simulink model "ConsolidatedModelV9"  (R2022a)
settings: Solver=VariableStepAuto  StartTime=0.0  StopTime=10.0  RelTol=1e-3
undefined symbols (not defined in the file or in its folder): s0
libraries: commblkcod2 x15, commchan3 x12, commdigbbndpm3 x12, simulink x9, commsink2 x6, commdigbbndam3 x6, rllib x3
settings Model: Creator=yangz  LastModifiedBy=yangz

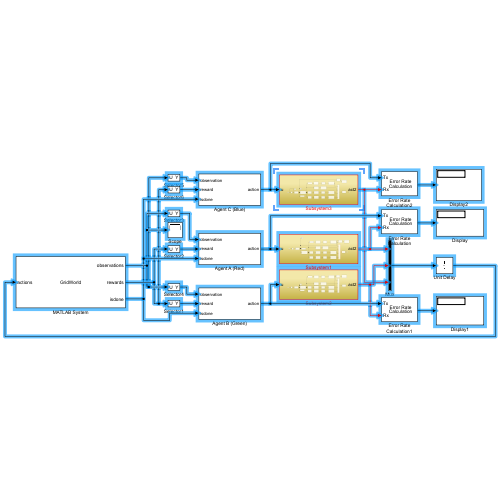
[thumbnail: Simulink's stored preview of the top-level diagram]
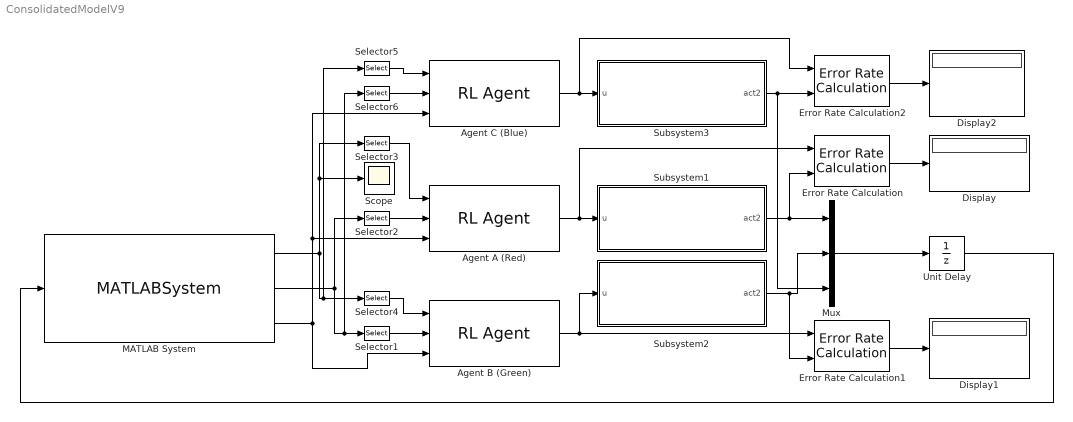
== system ConsolidatedModelV9 ==
  Agent A (Red) : rllib/RL Agent  Agent=agentA  ExternalActionAsInput=off  ProvideLastAction=off  ProvideCumRwd=off  TreatAsDirectFeedthrough=on  UseStrictObservationDataTypes=off
  Agent B (Green) : rllib/RL Agent  Agent=agentB  ExternalActionAsInput=off  ProvideLastAction=off  ProvideCumRwd=off  TreatAsDirectFeedthrough=on  UseStrictObservationDataTypes=off
  Agent C (Blue) : rllib/RL Agent  Agent=agentC  ExternalActionAsInput=off  ProvideLastAction=off  ProvideCumRwd=off  TreatAsDirectFeedthrough=on  UseStrictObservationDataTypes=off
  Display : Display
  Display1 : Display
  Display2 : Display
  Error Rate Calculation : commsink2/Error Rate Calculation  N=0  st_delay=0  cp_mode=Entire frame  subframe=[]  PMode=Port  WsName=ErrorVec  RsMode2=off  stop=off  numErr=100  maxBits=1e6
  Error Rate Calculation1 : commsink2/Error Rate Calculation  N=0  st_delay=0  cp_mode=Entire frame  subframe=[]  PMode=Port  WsName=ErrorVec  RsMode2=off  stop=off  numErr=100  maxBits=1e6
  Error Rate Calculation2 : commsink2/Error Rate Calculation  N=0  st_delay=0  cp_mode=Entire frame  subframe=[]  PMode=Port  WsName=ErrorVec  RsMode2=off  stop=off  numErr=100  maxBits=1e6
  MATLAB System : MATLABSystem  System=GridWorld  InitialStates=s0  Obstacles=obsMat  MaxStepCount=maxsteps  SimulateUsing=Interpreted execution
      mask Type: GridWorld
      mask Display:
      | disp('GridWorld');
      | port_label('input',1,'actions');
      | port_label('output',1,'observations');
      | port_label('output',2,'rewards');
      | port_label('output',3,'isdone');
  Mux : Mux  Inputs=3
  Scope : Scope
  Selector1 : Selector  InputPortWidth=3  IndexOptions=Index vector (dialog)  Indices=2  OutputSizes=1
  Selector2 : Selector  InputPortWidth=3  IndexOptions=Index vector (dialog)  Indices=1  OutputSizes=1
  Selector3 : Selector  NumberOfDimensions=4  InputPortWidth=3  IndexOptions=Select all,Select all,Select all,Index vector (dialog)  Indices=1,1,1,1  OutputSizes=1,1,1,1
  Selector4 : Selector  NumberOfDimensions=4  InputPortWidth=3  IndexOptions=Select all,Select all,Select all,Index vector (dialog)  Indices=1,1,1,2  OutputSizes=1,1,1,1
  Selector5 : Selector  NumberOfDimensions=4  InputPortWidth=3  IndexOptions=Select all,Select all,Select all,Index vector (dialog)  Indices=1,1,1,3  OutputSizes=1,1,1,1
  Selector6 : Selector  InputPortWidth=3  IndexOptions=Index vector (dialog)  Indices=3  OutputSizes=1
  Subsystem1 : Subsystem
  Subsystem2 : Subsystem
  Subsystem3 : Subsystem
  Unit Delay : UnitDelay  SampleTime=-1  HasFrameUpgradeWarning=on
  wires:
  Agent C (Blue)/1 -> Error Rate Calculation2/1, Subsystem3/1(u)
  Mux/1 -> Unit Delay/1
  MATLAB System/1 -> Selector4/1, Selector5/1, Scope/1, Selector3/1
  MATLAB System/3 -> Agent B (Green)/3, Agent A (Red)/3, Agent C (Blue)/3
  MATLAB System/2 -> Selector1/1, Selector6/1, Selector2/1
  Subsystem3/1(act2) -> Mux/3, Error Rate Calculation2/2
  Selector5/1 -> Agent C (Blue)/1
  Error Rate Calculation/1 -> Display/1
  Agent B (Green)/1 -> Subsystem2/1(u), Error Rate Calculation1/1
  Agent A (Red)/1 -> Subsystem1/1(u), Error Rate Calculation/1
  Subsystem2/1(act2) -> Mux/2, Error Rate Calculation1/2
  Subsystem1/1(act2) -> Mux/1, Error Rate Calculation/2
  Selector1/1 -> Agent B (Green)/2
  Selector6/1 -> Agent C (Blue)/2
  Selector4/1 -> Agent B (Green)/1
  Error Rate Calculation2/1 -> Display2/1
  Unit Delay/1 -> MATLAB System/1
  Selector3/1 -> Agent A (Red)/1
  Selector2/1 -> Agent A (Red)/2
  Error Rate Calculation1/1 -> Display1/1

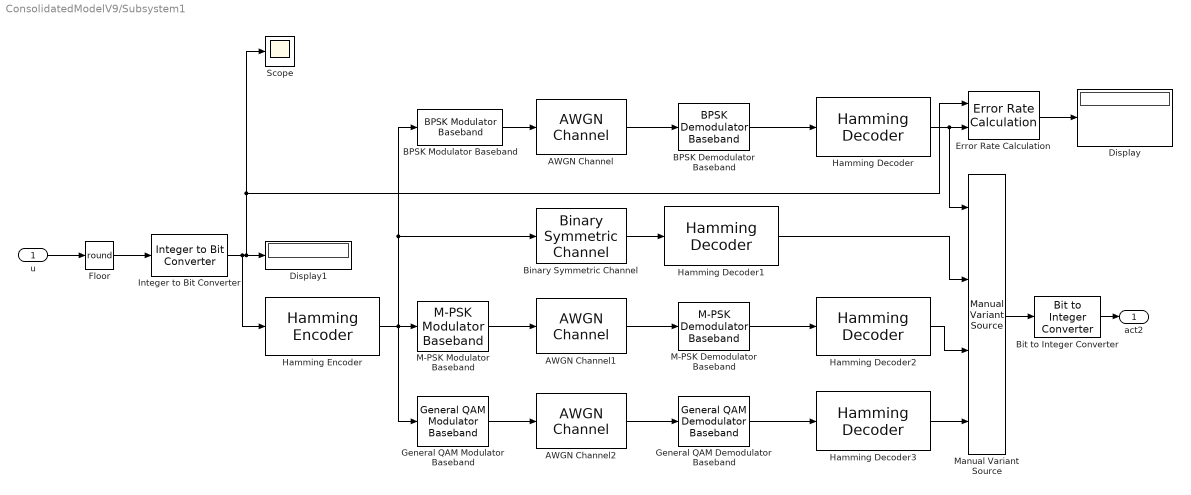
== system ConsolidatedModelV9/Subsystem1 ==
  u : Inport
  AWGN Channel : commchan3/AWGN Channel  InputProcessing=Columns as channels (frame based)  seed=67  noiseMode="Signal to noise ratio  (SNR)"  EbNodB=10  EsNodB=10  SNRdB=10  bitsPerSym=1  Ps=1  Tsym=1  variance=1
  AWGN Channel1 : commchan3/AWGN Channel  InputProcessing=Columns as channels (frame based)  seed=67  noiseMode="Signal to noise ratio  (SNR)"  EbNodB=10  EsNodB=10  SNRdB=10  bitsPerSym=1  Ps=1  Tsym=1  variance=1
  AWGN Channel2 : commchan3/AWGN Channel  InputProcessing=Columns as channels (frame based)  seed=67  noiseMode="Signal to noise ratio  (SNR)"  EbNodB=10  EsNodB=10  SNRdB=10  bitsPerSym=1  Ps=1  Tsym=1  variance=1
  BPSK Demodulator Baseband : commdigbbndpm3/BPSK Demodulator Baseband  DecType=Hard decision  VarSource=Dialog  Variance=1  Ph=0  outDtype=Inherit via internal rule  derotateFactorWordLen=16  derotateFactorDataTypeStr=Inherit: Same word length as input  derotateFactorLastDataTypeStr=Inherit: Same word length as input
  BPSK Modulator Baseband : commdigbbndpm3/BPSK Modulator Baseband  Ph=0  outDtype=double  outWordLen=16  outUDDataType=sfix(16)  outFracLenMode=Best precision  outFracLen=15  outDataTypeStr=double  outLastDataTypeStr=double
  Binary Symmetric Channel : commchan3/Binary Symmetric Channel  ErrorProbability=0.05  ErrorVectorOutputPort=off  OutputDataType=double  OutputDataTypeSL=double  Seed=71  SimulateUsing=Code generation
      settings: SourceProductBaseCode=CM
  Bit to Integer Converter : simulink/Logic and Bit Operations/Bit to Integer Converter  nbits=4  bitOrder=MSB first  signedOutputValues=Unsigned  outDtype=Inherit via internal rule  outDtypeSigned=Inherit via internal rule
      settings: SourceProductBaseCode=SL
  Display : Display
  Display1 : Display
  Error Rate Calculation : commsink2/Error Rate Calculation  N=0  st_delay=0  cp_mode=Entire frame  subframe=[]  PMode=Port  WsName=ErrorVec  RsMode2=off  stop=off  numErr=100  maxBits=1e6
  Floor : Rounding  Operator=round
  General QAM Demodulator Baseband : commdigbbndam3/General QAM Demodulator Baseband  SigCon=[exp(2*pi*1i*[0:7]/8)]  OutType=Integer  DecType=Hard decision  VarSource=Dialog  Variance=1  outDtypeBit=Inherit via internal rule  outDtype=Inherit via internal rule  roundingMode=Floor  overflowMode=Wrap  OvFlMode=off  OvFlModeLastStrValue=off  sigConstWordLen=16  sigConstDataTypeStr=Inherit: Same word length as input  sigConstLastDataTypeStr=Inherit: Same word length as input  accum1WordLen=32  accum1FracLen=30  prodInWordLen=32  prodInFracLen=30  prodInDataTypeStr=Inherit: Same as accumulator 1  prodInLastDataTypeStr=Inherit: Same as accumulator 1  prodOutWordLen=32  prodOutFracLen=30  accum2WordLen=32  accum2FracLen=30  accum3WordLen=32  accum3FracLen=30  nsiWordLen=32  nsiFracLen=30  nsiDataTypeStr=Inherit: Same as accumulator 3  nsiLastDataTypeStr=Inherit: Same as accumulator 3  invn0WordLen=16  invn0FracLen=8  invn0DataTypeStr=Inherit: Same word length as input  invn0LastDataTypeStr=Inherit: Same word length as input  outputWordLen=32  outputFracLen=30
      settings: SourceProductBaseCode=CM
  General QAM Modulator Baseband : commdigbbndam3/General QAM Modulator Baseband  SigCon=[exp(2*pi*1i*[0:7]/8)]  outDtype=double  outWordLen=16  outUDDataType=sfix(16)  outFracLenMode=Best precision  outFracLen=15  outDataTypeStr=double  outLastDataTypeStr=double
      settings: SourceProductBaseCode=CM
  Hamming Decoder{,1..3} (4 alike) : commblkcod2/Hamming Decoder  n=7  k=4
      settings: SourceProductBaseCode=CM
  Hamming Encoder : commblkcod2/Hamming Encoder  n=7  k=4
      settings: SourceProductBaseCode=CM
  Integer to Bit Converter : simulink/Logic and Bit Operations/Integer to Bit Converter  nbits=4  signedInputValues=Unsigned  bitOrder=MSB first  outDtype=Inherit via internal rule
      settings: SourceProductBaseCode=SL
  M-PSK Demodulator Baseband : commdigbbndpm3/M-PSK Demodulator Baseband  M=8  OutType=Integer  DecType=Hard decision  VarSource=Dialog  Variance=1  Dec=Gray  Mapping=[0:7]  Ph=pi/8  outDtype1=Inherit via internal rule  outDtype2=Inherit via internal rule  derotateFactorWordLen=16  derotateFactorDataTypeStr=Inherit: Same word length as input  derotateFactorLastDataTypeStr=Inherit: Same word length as input
  M-PSK Modulator Baseband : commdigbbndpm3/M-PSK Modulator Baseband  M=8  InType=Integer  Enc=Gray  Mapping=[0:7]  Ph=pi/8  outDtype=double  outWordLen=16  outUDDataType=sfix(16)  outFracLenMode=Best precision  outFracLen=15  outDataTypeStr=double  outLastDataTypeStr=double
  Manual Variant Source : simulink/Signal Routing/Manual Variant Source  NumChoices=4  LabelModeActiveChoice=V_3
  Scope : Scope
  act2 : Outport
  wires:
  Binary Symmetric Channel/1 -> Hamming Decoder1/1
  AWGN Channel1/1 -> M-PSK Demodulator Baseband/1
  BPSK Demodulator Baseband/1 -> Hamming Decoder/1
  M-PSK Demodulator Baseband/1 -> Hamming Decoder2/1
  M-PSK Modulator Baseband/1 -> AWGN Channel1/1
  Error Rate Calculation/1 -> Display/1
  AWGN Channel/1 -> BPSK Demodulator Baseband/1
  BPSK Modulator Baseband/1 -> AWGN Channel/1
  Bit to Integer Converter/1 -> act2/1
  General QAM Modulator Baseband/1 -> AWGN Channel2/1
  Floor/1 -> Integer to Bit Converter/1
  u/1 -> Floor/1
  Hamming Decoder1/1 -> Manual Variant Source/2
  AWGN Channel2/1 -> General QAM Demodulator Baseband/1
  Hamming Decoder2/1 -> Manual Variant Source/3
  Hamming Decoder3/1 -> Manual Variant Source/4
  General QAM Demodulator Baseband/1 -> Hamming Decoder3/1
  Hamming Decoder/1 -> Error Rate Calculation/2, Manual Variant Source/1
  Hamming Encoder/1 -> BPSK Modulator Baseband/1, Binary Symmetric Channel/1, M-PSK Modulator Baseband/1, General QAM Modulator Baseband/1
  Integer to Bit Converter/1 -> Error Rate Calculation/1, Scope/1, Display1/1, Hamming Encoder/1
  Manual Variant Source/1 -> Bit to Integer Converter/1

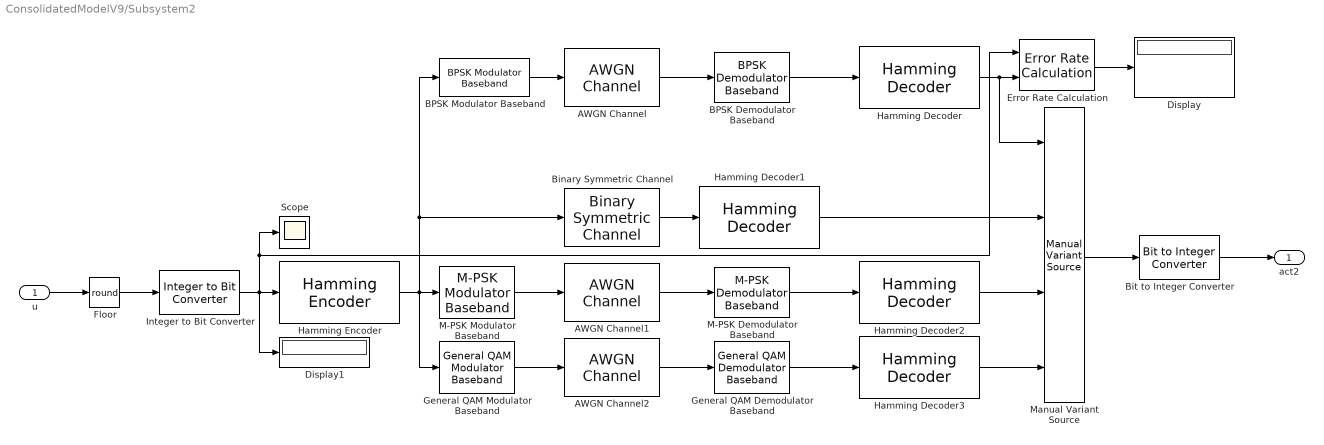
== system ConsolidatedModelV9/Subsystem2 ==
  u : Inport
  AWGN Channel : commchan3/AWGN Channel  InputProcessing=Columns as channels (frame based)  seed=67  noiseMode="Signal to noise ratio  (SNR)"  EbNodB=10  EsNodB=10  SNRdB=10  bitsPerSym=1  Ps=1  Tsym=1  variance=1
  AWGN Channel1 : commchan3/AWGN Channel  InputProcessing=Columns as channels (frame based)  seed=67  noiseMode="Signal to noise ratio  (SNR)"  EbNodB=10  EsNodB=10  SNRdB=10  bitsPerSym=1  Ps=1  Tsym=1  variance=1
  AWGN Channel2 : commchan3/AWGN Channel  InputProcessing=Columns as channels (frame based)  seed=67  noiseMode="Signal to noise ratio  (SNR)"  EbNodB=10  EsNodB=10  SNRdB=10  bitsPerSym=1  Ps=1  Tsym=1  variance=1
  BPSK Demodulator Baseband : commdigbbndpm3/BPSK Demodulator Baseband  DecType=Hard decision  VarSource=Dialog  Variance=1  Ph=0  outDtype=Inherit via internal rule  derotateFactorWordLen=16  derotateFactorDataTypeStr=Inherit: Same word length as input  derotateFactorLastDataTypeStr=Inherit: Same word length as input
  BPSK Modulator Baseband : commdigbbndpm3/BPSK Modulator Baseband  Ph=0  outDtype=double  outWordLen=16  outUDDataType=sfix(16)  outFracLenMode=Best precision  outFracLen=15  outDataTypeStr=double  outLastDataTypeStr=double
  Binary Symmetric Channel : commchan3/Binary Symmetric Channel  ErrorProbability=0.05  ErrorVectorOutputPort=off  OutputDataType=double  OutputDataTypeSL=double  Seed=71  SimulateUsing=Code generation
      settings: SourceProductBaseCode=CM
  Bit to Integer Converter : simulink/Logic and Bit Operations/Bit to Integer Converter  nbits=4  bitOrder=MSB first  signedOutputValues=Unsigned  outDtype=Inherit via internal rule  outDtypeSigned=Inherit via internal rule
      settings: SourceProductBaseCode=SL
  Display : Display
  Display1 : Display
  Error Rate Calculation : commsink2/Error Rate Calculation  N=0  st_delay=0  cp_mode=Entire frame  subframe=[]  PMode=Port  WsName=ErrorVec  RsMode2=off  stop=off  numErr=100  maxBits=1e6
  Floor : Rounding  Operator=round
  General QAM Demodulator Baseband : commdigbbndam3/General QAM Demodulator Baseband  SigCon=[exp(2*pi*1i*[0:7]/8)]  OutType=Integer  DecType=Hard decision  VarSource=Dialog  Variance=1  outDtypeBit=Inherit via internal rule  outDtype=Inherit via internal rule  roundingMode=Floor  overflowMode=Wrap  OvFlMode=off  OvFlModeLastStrValue=off  sigConstWordLen=16  sigConstDataTypeStr=Inherit: Same word length as input  sigConstLastDataTypeStr=Inherit: Same word length as input  accum1WordLen=32  accum1FracLen=30  prodInWordLen=32  prodInFracLen=30  prodInDataTypeStr=Inherit: Same as accumulator 1  prodInLastDataTypeStr=Inherit: Same as accumulator 1  prodOutWordLen=32  prodOutFracLen=30  accum2WordLen=32  accum2FracLen=30  accum3WordLen=32  accum3FracLen=30  nsiWordLen=32  nsiFracLen=30  nsiDataTypeStr=Inherit: Same as accumulator 3  nsiLastDataTypeStr=Inherit: Same as accumulator 3  invn0WordLen=16  invn0FracLen=8  invn0DataTypeStr=Inherit: Same word length as input  invn0LastDataTypeStr=Inherit: Same word length as input  outputWordLen=32  outputFracLen=30
      settings: SourceProductBaseCode=CM
  General QAM Modulator Baseband : commdigbbndam3/General QAM Modulator Baseband  SigCon=[exp(2*pi*1i*[0:7]/8)]  outDtype=double  outWordLen=16  outUDDataType=sfix(16)  outFracLenMode=Best precision  outFracLen=15  outDataTypeStr=double  outLastDataTypeStr=double
      settings: SourceProductBaseCode=CM
  Hamming Decoder{,1..3} (4 alike) : commblkcod2/Hamming Decoder  n=7  k=4
      settings: SourceProductBaseCode=CM
  Hamming Encoder : commblkcod2/Hamming Encoder  n=7  k=4
      settings: SourceProductBaseCode=CM
  Integer to Bit Converter : simulink/Logic and Bit Operations/Integer to Bit Converter  nbits=4  signedInputValues=Unsigned  bitOrder=MSB first  outDtype=Inherit via internal rule
      settings: SourceProductBaseCode=SL
  M-PSK Demodulator Baseband : commdigbbndpm3/M-PSK Demodulator Baseband  M=8  OutType=Integer  DecType=Hard decision  VarSource=Dialog  Variance=1  Dec=Gray  Mapping=[0:7]  Ph=pi/8  outDtype1=Inherit via internal rule  outDtype2=Inherit via internal rule  derotateFactorWordLen=16  derotateFactorDataTypeStr=Inherit: Same word length as input  derotateFactorLastDataTypeStr=Inherit: Same word length as input
  M-PSK Modulator Baseband : commdigbbndpm3/M-PSK Modulator Baseband  M=8  InType=Integer  Enc=Gray  Mapping=[0:7]  Ph=pi/8  outDtype=double  outWordLen=16  outUDDataType=sfix(16)  outFracLenMode=Best precision  outFracLen=15  outDataTypeStr=double  outLastDataTypeStr=double
  Manual Variant Source : simulink/Signal Routing/Manual Variant Source  NumChoices=4  LabelModeActiveChoice=V_3
  Scope : Scope
  act2 : Outport
  wires:
  Manual Variant Source/1 -> Bit to Integer Converter/1
  General QAM Modulator Baseband/1 -> AWGN Channel2/1
  Hamming Decoder1/1 -> Manual Variant Source/2
  Hamming Decoder2/1 -> Manual Variant Source/3
  Hamming Decoder3/1 -> Manual Variant Source/4
  AWGN Channel2/1 -> General QAM Demodulator Baseband/1
  General QAM Demodulator Baseband/1 -> Hamming Decoder3/1
  Floor/1 -> Integer to Bit Converter/1
  M-PSK Demodulator Baseband/1 -> Hamming Decoder2/1
  u/1 -> Floor/1
  Bit to Integer Converter/1 -> act2/1
  M-PSK Modulator Baseband/1 -> AWGN Channel1/1
  Error Rate Calculation/1 -> Display/1
  AWGN Channel/1 -> BPSK Demodulator Baseband/1
  BPSK Demodulator Baseband/1 -> Hamming Decoder/1
  BPSK Modulator Baseband/1 -> AWGN Channel/1
  Binary Symmetric Channel/1 -> Hamming Decoder1/1
  AWGN Channel1/1 -> M-PSK Demodulator Baseband/1
  Hamming Encoder/1 -> Binary Symmetric Channel/1, BPSK Modulator Baseband/1, M-PSK Modulator Baseband/1, General QAM Modulator Baseband/1
  Integer to Bit Converter/1 -> Scope/1, Error Rate Calculation/1, Display1/1, Hamming Encoder/1
  Hamming Decoder/1 -> Manual Variant Source/1, Error Rate Calculation/2

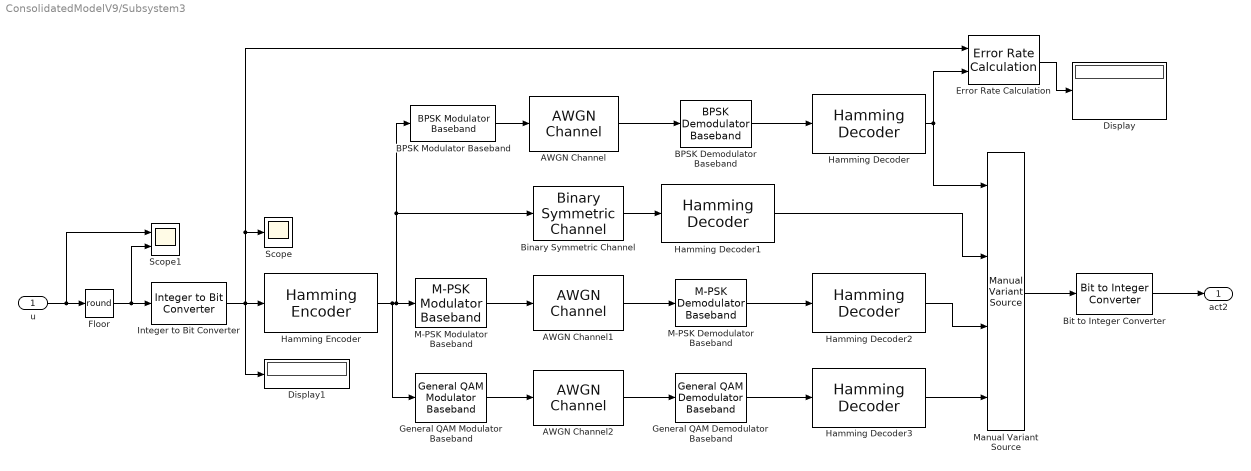
== system ConsolidatedModelV9/Subsystem3 ==
  u : Inport
  AWGN Channel : commchan3/AWGN Channel  InputProcessing=Columns as channels (frame based)  seed=67  noiseMode="Signal to noise ratio  (SNR)"  EbNodB=10  EsNodB=10  SNRdB=10  bitsPerSym=1  Ps=1  Tsym=1  variance=1
  AWGN Channel1 : commchan3/AWGN Channel  InputProcessing=Columns as channels (frame based)  seed=67  noiseMode="Signal to noise ratio  (SNR)"  EbNodB=10  EsNodB=10  SNRdB=10  bitsPerSym=1  Ps=1  Tsym=1  variance=1
  AWGN Channel2 : commchan3/AWGN Channel  InputProcessing=Columns as channels (frame based)  seed=67  noiseMode="Signal to noise ratio  (SNR)"  EbNodB=10  EsNodB=10  SNRdB=10  bitsPerSym=1  Ps=1  Tsym=1  variance=1
  BPSK Demodulator Baseband : commdigbbndpm3/BPSK Demodulator Baseband  DecType=Hard decision  VarSource=Dialog  Variance=1  Ph=0  outDtype=Inherit via internal rule  derotateFactorWordLen=16  derotateFactorDataTypeStr=Inherit: Same word length as input  derotateFactorLastDataTypeStr=Inherit: Same word length as input
  BPSK Modulator Baseband : commdigbbndpm3/BPSK Modulator Baseband  Ph=0  outDtype=double  outWordLen=16  outUDDataType=sfix(16)  outFracLenMode=Best precision  outFracLen=15  outDataTypeStr=double  outLastDataTypeStr=double
  Binary Symmetric Channel : commchan3/Binary Symmetric Channel  ErrorProbability=0.05  ErrorVectorOutputPort=off  OutputDataType=double  OutputDataTypeSL=double  Seed=67  SimulateUsing=Code generation
      settings: SourceProductBaseCode=CM
  Bit to Integer Converter : simulink/Logic and Bit Operations/Bit to Integer Converter  nbits=4  bitOrder=MSB first  signedOutputValues=Unsigned  outDtype=Inherit via internal rule  outDtypeSigned=Inherit via internal rule
      settings: SourceProductBaseCode=SL
  Display : Display
  Display1 : Display
  Error Rate Calculation : commsink2/Error Rate Calculation  N=0  st_delay=0  cp_mode=Entire frame  subframe=[]  PMode=Port  WsName=ErrorVec  RsMode2=off  stop=off  numErr=100  maxBits=1e6
  Floor : Rounding  Operator=round
  General QAM Demodulator Baseband : commdigbbndam3/General QAM Demodulator Baseband  SigCon=[exp(2*pi*1i*[0:7]/8)]  OutType=Integer  DecType=Hard decision  VarSource=Dialog  Variance=1  outDtypeBit=Inherit via internal rule  outDtype=Inherit via internal rule  roundingMode=Floor  overflowMode=Wrap  OvFlMode=off  OvFlModeLastStrValue=off  sigConstWordLen=16  sigConstDataTypeStr=Inherit: Same word length as input  sigConstLastDataTypeStr=Inherit: Same word length as input  accum1WordLen=32  accum1FracLen=30  prodInWordLen=32  prodInFracLen=30  prodInDataTypeStr=Inherit: Same as accumulator 1  prodInLastDataTypeStr=Inherit: Same as accumulator 1  prodOutWordLen=32  prodOutFracLen=30  accum2WordLen=32  accum2FracLen=30  accum3WordLen=32  accum3FracLen=30  nsiWordLen=32  nsiFracLen=30  nsiDataTypeStr=Inherit: Same as accumulator 3  nsiLastDataTypeStr=Inherit: Same as accumulator 3  invn0WordLen=16  invn0FracLen=8  invn0DataTypeStr=Inherit: Same word length as input  invn0LastDataTypeStr=Inherit: Same word length as input  outputWordLen=32  outputFracLen=30
      settings: SourceProductBaseCode=CM
  General QAM Modulator Baseband : commdigbbndam3/General QAM Modulator Baseband  SigCon=[exp(2*pi*1i*[0:7]/8)]  outDtype=double  outWordLen=16  outUDDataType=sfix(16)  outFracLenMode=Best precision  outFracLen=15  outDataTypeStr=double  outLastDataTypeStr=double
      settings: SourceProductBaseCode=CM
  Hamming Decoder{,1..3} (4 alike) : commblkcod2/Hamming Decoder  n=7  k=4
      settings: SourceProductBaseCode=CM
  Hamming Encoder : commblkcod2/Hamming Encoder  n=7  k=4
      settings: SourceProductBaseCode=CM
  Integer to Bit Converter : simulink/Logic and Bit Operations/Integer to Bit Converter  nbits=4  signedInputValues=Unsigned  bitOrder=MSB first  outDtype=Inherit via internal rule
      settings: SourceProductBaseCode=SL
  M-PSK Demodulator Baseband : commdigbbndpm3/M-PSK Demodulator Baseband  M=8  OutType=Integer  DecType=Hard decision  VarSource=Dialog  Variance=1  Dec=Gray  Mapping=[0:7]  Ph=pi/8  outDtype1=Inherit via internal rule  outDtype2=Inherit via internal rule  derotateFactorWordLen=16  derotateFactorDataTypeStr=Inherit: Same word length as input  derotateFactorLastDataTypeStr=Inherit: Same word length as input
  M-PSK Modulator Baseband : commdigbbndpm3/M-PSK Modulator Baseband  M=8  InType=Integer  Enc=Gray  Mapping=[0:7]  Ph=pi/8  outDtype=double  outWordLen=16  outUDDataType=sfix(16)  outFracLenMode=Best precision  outFracLen=15  outDataTypeStr=double  outLastDataTypeStr=double
  Manual Variant Source : simulink/Signal Routing/Manual Variant Source  NumChoices=4  LabelModeActiveChoice=V_3
  Scope : Scope
  Scope1 : Scope  NumInputPorts=2
  act2 : Outport
  wires:
  Hamming Decoder1/1 -> Manual Variant Source/2
  General QAM Modulator Baseband/1 -> AWGN Channel2/1
  Manual Variant Source/1 -> Bit to Integer Converter/1
  Hamming Decoder3/1 -> Manual Variant Source/4
  General QAM Demodulator Baseband/1 -> Hamming Decoder3/1
  M-PSK Modulator Baseband/1 -> AWGN Channel1/1
  AWGN Channel2/1 -> General QAM Demodulator Baseband/1
  Bit to Integer Converter/1 -> act2/1
  Floor/1 -> Scope1/2, Integer to Bit Converter/1
  Error Rate Calculation/1 -> Display/1
  AWGN Channel/1 -> BPSK Demodulator Baseband/1
  BPSK Demodulator Baseband/1 -> Hamming Decoder/1
  BPSK Modulator Baseband/1 -> AWGN Channel/1
  M-PSK Demodulator Baseband/1 -> Hamming Decoder2/1
  Hamming Decoder2/1 -> Manual Variant Source/3
  Binary Symmetric Channel/1 -> Hamming Decoder1/1
  AWGN Channel1/1 -> M-PSK Demodulator Baseband/1
  u/1 -> Scope1/1, Floor/1
  Integer to Bit Converter/1 -> Scope/1, Error Rate Calculation/1, Display1/1, Hamming Encoder/1
  Hamming Encoder/1 -> Binary Symmetric Channel/1, BPSK Modulator Baseband/1, M-PSK Modulator Baseband/1, General QAM Modulator Baseband/1
  Hamming Decoder/1 -> Error Rate Calculation/2, Manual Variant Source/1
